simulink model "LQR_simulation"  (R2023a)
settings: Solver=FixedStepAuto  StartTime=0.0  StopTime=100  FixedStep=out_rate  RelTol=1e-3
InitFcn:
  | LQR_init
values from neighbouring files (symbols this model uses):
  C = [1 0 0 0;     0 1 0 0]    [LQR_init.m]
  dt = 0.001    [LQR_init.m]
  dtheta_0_real = dtheta_0+std_dev.dtheta_0*rand(1,1)    [LQR_init.m]
  dz_0_real = dz_0+std_dev.dz_0*randn(1,1)    [LQR_init.m]
  fa_w = 0    [LQR_init.m]
  fm_w = s_param.g*s_param.m    [LQR_init.m]
  K_a_lqr = - lqr(A_a,B_a,Q_a_lqr,R_a_lqr)    [LQR_init.m]
  K_lqr = - lqr(A,B,Q_lqr,R_lqr)    [LQR_init.m]
  Km1 = 1.1    [LQR_init.m]
  Km1_real = Km1 + std_dev_Km*randn(1,1)    [LQR_init.m]
  Km2 = 1.1    [LQR_init.m]
  Km2_real = Km2 + std_dev_Km*randn(1,1)    [LQR_init.m]
  m_treshold = 5    [LQR_init.m]
  out_rate = 0.001    [LQR_init.m]
  P_0 = blkdiag(std_dev.z_0^2, std_dev.theta_0^2, std_dev.dz_0^2, std_dev.dtheta_0^2)    [LQR_init.m]
  Q = blkdiag(std_dev.fm^2, std_dev.fa^2)    [LQR_init.m]
  R = blkdiag(std_dev.y1^2, std_dev.y2^2)    [LQR_init.m]
  T1 = 0.05    [LQR_init.m]
  T1_real = T1 + std_dev_T*randn(1,1)    [LQR_init.m]
  T2 = 0.15    [LQR_init.m]
  T2_real = T2 + std_dev_T*randn(1,1)    [LQR_init.m]
  theta_0_real = theta_0+std_dev.theta_0*randn(1,1)    [LQR_init.m]
  theta_w = 0    [LQR_init.m]
  Tm1 = 1    [LQR_init.m]
  Tm1_real = Tm1 + std_dev_Tm*randn(1,1)    [LQR_init.m]
  Tm2 = 1    [LQR_init.m]
  Tm2_real = Tm2 + std_dev_Tm*randn(1,1)    [LQR_init.m]
  U_mean = [0; 0]    [LQR_init.m]
  x_0 = [z_0; theta_0; dz_0; dtheta_0]    [LQR_init.m]
  x_a_w = [0;0;x_w]    [LQR_init.m]
  x_w = [z_w; theta_w; dz_w; dtheta_w]    [LQR_init.m]
  z_0_real = z_0+std_dev.z_0*randn(1,1)    [LQR_init.m]
  z_w = 400    [LQR_init.m]
undefined symbols (not defined in the file or in its folder): Kf, s_param, std_dev, Ts
libraries: simulink x4
settings Model: Creator=franc  LastModifiedBy=rvitt

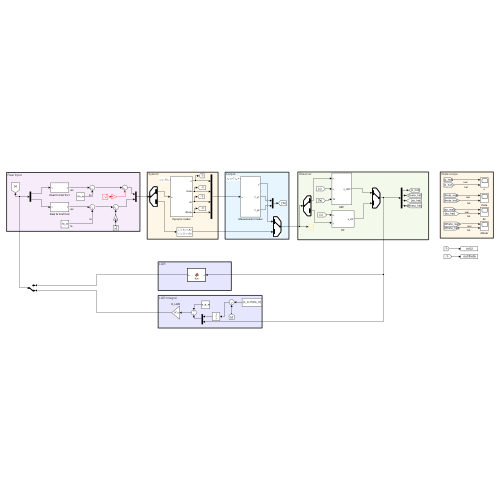
[thumbnail: Simulink's stored preview of the top-level diagram]
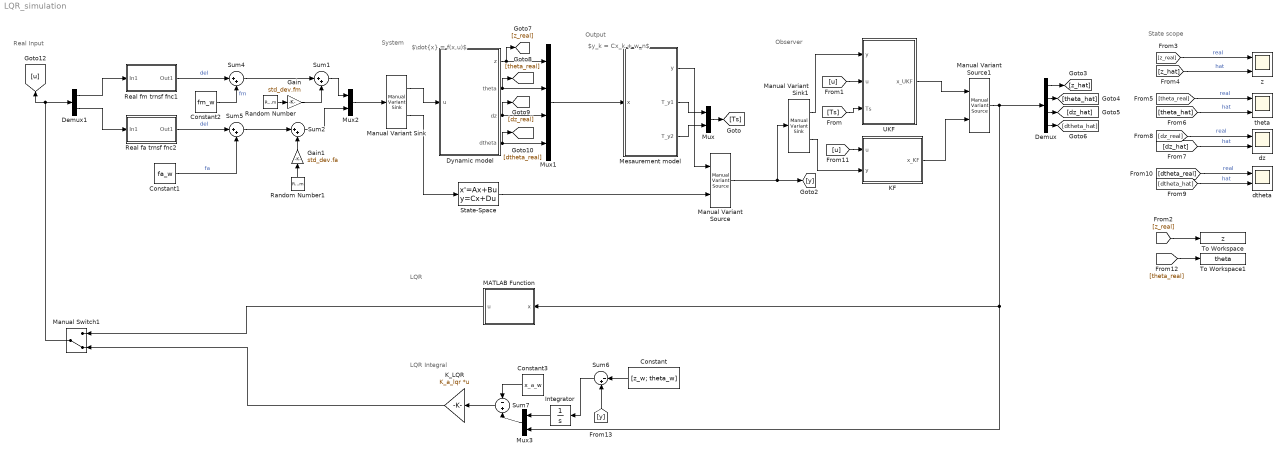
== system LQR_simulation ==
  note: State scope
  note: LQR Integral
  note: LQR
  note: Real Input
  note: Observer
  note: $y_k = Cx_k + w_n$
  note: Output
  note: $\dot{x} = f(x,u)$
  note: System
  Constant : Constant  Value=[z_w; theta_w]
  Constant1 : Constant  Value=fa_w
  Constant2 : Constant  Value=fm_w
  Constant3 : Constant  Value=x_a_w
  Demux : Demux
  Demux1 : Demux  Outputs=2
  Dynamic model : Subsystem
  Gain : Gain  Gain=std_dev.fm
  Gain1 : Gain  Gain=std_dev.fa
  Integrator : Integrator
  KF : Subsystem
  K_LQR : Gain  Gain=K_a_lqr  Multiplication=Matrix(K*u)
  MATLAB Function : MATLAB Function  TreatAsAtomicUnit=on
  Manual Variant Sink : simulink/Signal Routing/Manual Variant Sink  NumChoices=2  LabelModeActiveChoice=V_1
  Manual Variant Sink1 : simulink/Signal Routing/Manual Variant Sink  NumChoices=2  LabelModeActiveChoice=V_1
  Manual Variant Source : simulink/Signal Routing/Manual Variant Source  NumChoices=2  LabelModeActiveChoice=V_1
  Manual Variant Source1 : simulink/Signal Routing/Manual Variant Source  NumChoices=2  LabelModeActiveChoice=V_1
  Manual Switch1 : ManualSwitch  CurrentSetting=0
  Mesaurement model : Subsystem
  Mux : Mux  Inputs=2
  Mux1 : Mux
  Mux2 : Mux  Inputs=2
  Mux3 : Mux  Inputs=2
  Random Number : RandomNumber  SampleTime=out_rate
  Random Number1 : RandomNumber  SampleTime=out_rate
  Real fa trnsf fnc2 : Subsystem
  Real fm trnsf fnc1 : Subsystem
  State-Space : StateSpace  InitialCondition=0
  Sum{1..2,4..5} (4 alike) : Sum  Inputs=|++
  Sum6 : Sum  Inputs=|-+
  Sum7 : Sum  Inputs=-|+
  To Workspace : ToWorkspace  VariableName=z  SaveFormat=Timeseries  SampleTime=-1
  To Workspace1 : ToWorkspace  VariableName=theta  SaveFormat=Timeseries  SampleTime=-1
  UKF : Subsystem
  dtheta : Scope  NumInputPorts=2
  dz : Scope  NumInputPorts=2
  theta : Scope  NumInputPorts=2
  z : Scope  NumInputPorts=2
  wires:
  Mesaurement model/2(T_y1) -> Mux/1
  Mesaurement model/3(T_y2) -> Mux/2
  Mux/1 -> [Ts]
  [u] -> UKF/2(u)
  [Ts] -> UKF/3(Ts)
  UKF/1(x_UKF) -> Manual Variant Source1/1
  [z_real] -> z/1  "real"
  [z_hat] -> z/2  "hat"
  [theta_real] -> theta/1  "real"
  [theta_hat] -> theta/2  "hat"
  [dz_hat] -> dz/2  "hat"
  [dz_real] -> dz/1  "real"
  [dtheta_hat] -> dtheta/2  "hat"
  [dtheta_real] -> dtheta/1  "real"
  Mux1/1 -> Mesaurement model/1(x)
  Dynamic model/1(z) -> [z_real], Mux1/1
  Dynamic model/2(theta) -> Mux1/2, [theta_real]
  Dynamic model/3(dz) -> Mux1/3, [dz_real]
  Dynamic model/4(dtheta) -> Mux1/4, [dtheta_real]
  [u] -> KF/1(u)
  KF/1(x_KF) -> Manual Variant Source1/2
  Manual Variant Source1/1 -> MATLAB Function/1(x), Mux3/2, Demux/1
  Demux/1 -> [z_hat]
  Demux/2 -> [theta_hat]
  Demux/3 -> [dz_hat]
  Demux/4 -> [dtheta_hat]
  MATLAB Function/1(u) -> Manual Switch1/1
  Demux1/1 -> Real fm trnsf fnc1/1(In1)
  Sum1/1 -> Mux2/1
  Sum2/1 -> Mux2/2
  Gain/1 -> Sum1/2
  Gain1/1 -> Sum2/2
  Random Number/1 -> Gain/1
  Random Number1/1 -> Gain1/1
  Demux1/2 -> Real fa trnsf fnc2/1(In1)
  Real fm trnsf fnc1/1(Out1) -> Sum4/1  "del"
  Real fa trnsf fnc2/1(Out1) -> Sum5/1  "del"
  Sum4/1 -> Sum1/1
  Sum5/1 -> Sum2/1
  Constant2/1 -> Sum4/2  "fm"
  Constant1/1 -> Sum5/2  "fa"
  Manual Switch1/1 -> Demux1/1, [u]
  Constant/1 -> Sum6/1
  Mux3/1 -> Sum7/2
  Integrator/1 -> Mux3/1
  Sum6/1 -> Integrator/1
  [y] -> Sum6/2
  Mux2/1 -> Manual Variant Sink/1
  Manual Variant Sink/1 -> Dynamic model/1(u)
  Manual Variant Sink/2 -> State-Space/1
  Manual Variant Source/1 -> [y], Manual Variant Sink1/1
  Mesaurement model/1(y) -> Manual Variant Source/1
  State-Space/1 -> Manual Variant Source/2
  Manual Variant Sink1/1 -> UKF/1(y)
  Manual Variant Sink1/2 -> KF/2(y)
  Constant3/1 -> Sum7/1
  Sum7/1 -> K_LQR/1
  K_LQR/1 -> Manual Switch1/2
  [z_real] -> To Workspace/1
  [theta_real] -> To Workspace1/1

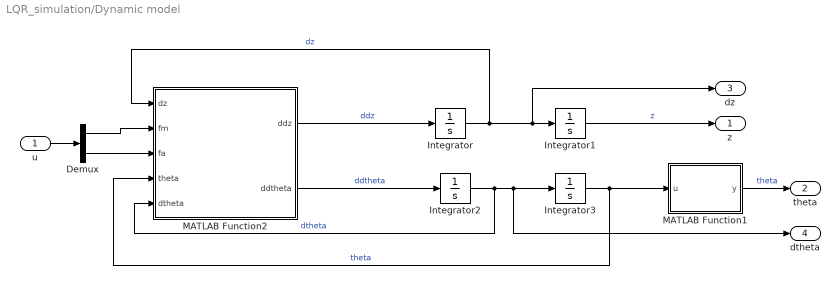
== system LQR_simulation/Dynamic model ==
  u : Inport
  Demux : Demux  Outputs=2
  Integrator : Integrator  InitialCondition=dz_0_real
  Integrator1 : Integrator  InitialCondition=z_0_real
  Integrator2 : Integrator  InitialCondition=dtheta_0_real
  Integrator3 : Integrator  InitialCondition=theta_0_real
  MATLAB Function1 : MATLAB Function  TreatAsAtomicUnit=on
  MATLAB Function2 : MATLAB Function  TreatAsAtomicUnit=on
  z : Outport
  theta : Outport  Port=2
  dz : Outport  Port=3
  dtheta : Outport  Port=4
  wires:
  Integrator3/1 -> MATLAB Function2/4(theta), MATLAB Function1/1(u)  "theta"
  Integrator2/1 -> dtheta/1, Integrator3/1, MATLAB Function2/5(dtheta)  "dtheta"
  MATLAB Function1/1(y) -> theta/1  "theta"
  Integrator1/1 -> z/1  "z"
  MATLAB Function2/2(ddtheta) -> Integrator2/1  "ddtheta"
  MATLAB Function2/1(ddz) -> Integrator/1  "ddz"
  Integrator/1 -> dz/1, Integrator1/1, MATLAB Function2/1(dz)  "dz"
  u/1 -> Demux/1
  Demux/2 -> MATLAB Function2/3(fa)
  Demux/1 -> MATLAB Function2/2(fm)

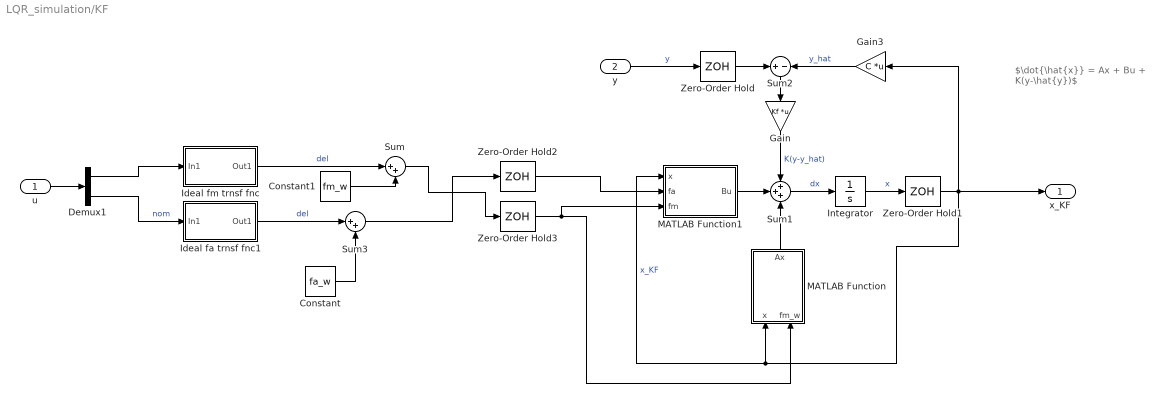
== system LQR_simulation/KF ==
  note: $\dot{\hat{x}} = Ax + Bu + K(y-\hat{y})$
  u : Inport
  y : Inport  Port=2
  Constant : Constant  Value=fa_w
  Constant1 : Constant  Value=fm_w
  Demux1 : Demux  Outputs=2
  Gain : Gain  Gain=Kf  Multiplication=Matrix(K*u)
  Gain3 : Gain  Gain=C  Multiplication=Matrix(K*u)
  Ideal fa trnsf fnc1 : Subsystem
  Ideal fm trnsf fnc : Subsystem
  Integrator : Integrator  InitialCondition=x_0
  MATLAB Function : MATLAB Function  TreatAsAtomicUnit=on
  MATLAB Function1 : MATLAB Function  TreatAsAtomicUnit=on
  Sum : Sum  Inputs=|++
  Sum1 : Sum  Inputs=+++
  Sum2 : Sum  Inputs=+|-
  Sum3 : Sum  Inputs=|++
  Zero-Order Hold{,1..3} (4 alike) : ZeroOrderHold  SampleTime=dt
  x_KF : Outport
  wires:
  y/1 -> Zero-Order Hold/1  "y"
  u/1 -> Demux1/1
  Gain3/1 -> Sum2/2  "y_hat"
  Sum1/1 -> Integrator/1  "dx"
  Sum2/1 -> Gain/1
  Gain/1 -> Sum1/1  "K(y-y_hat)"
  MATLAB Function1/1(Bu) -> Sum1/2
  Zero-Order Hold/1 -> Sum2/1
  Zero-Order Hold1/1 -> MATLAB Function1/1(x), MATLAB Function/1(x), Gain3/1, x_KF/1  "x_KF"
  Integrator/1 -> Zero-Order Hold1/1  "x"
  MATLAB Function/1(Ax) -> Sum1/3
  Zero-Order Hold2/1 -> MATLAB Function1/2(fa)
  Sum/1 -> Zero-Order Hold3/1
  Zero-Order Hold3/1 -> MATLAB Function1/3(fm), MATLAB Function/2(fm_w)
  Ideal fm trnsf fnc/1(Out1) -> Sum/1  "del"
  Constant1/1 -> Sum/2
  Demux1/1 -> Ideal fm trnsf fnc/1(In1)
  Ideal fa trnsf fnc1/1(Out1) -> Sum3/1  "del"
  Demux1/2 -> Ideal fa trnsf fnc1/1(In1)  "nom"
  Sum3/1 -> Zero-Order Hold2/1
  Constant/1 -> Sum3/2

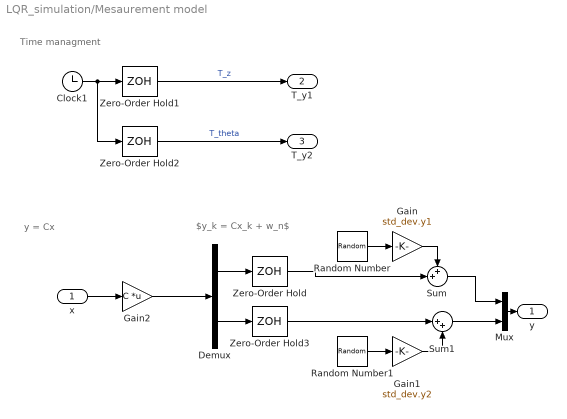
== system LQR_simulation/Mesaurement model ==
  note: $y_k = Cx_k + w_n$
  note: y = Cx
  note: Time managment
  x : Inport
  Clock1 : Clock
  Demux : Demux  Outputs=2
  Gain : Gain  Gain=std_dev.y1
  Gain1 : Gain  Gain=std_dev.y2
  Gain2 : Gain  Gain=C  Multiplication=Matrix(K*u)
  Mux : Mux  Inputs=2
  Random Number : RandomNumber  SampleTime=Ts.y1
  Random Number1 : RandomNumber  SampleTime=Ts.y2
  Sum : Sum  Inputs=++|
  Sum1 : Sum  Inputs=|++
  Zero-Order Hold : ZeroOrderHold  SampleTime=Ts.y1
  Zero-Order Hold1 : ZeroOrderHold  SampleTime=Ts.y1
  Zero-Order Hold2 : ZeroOrderHold  SampleTime=Ts.y2
  Zero-Order Hold3 : ZeroOrderHold  SampleTime=Ts.y2
  y : Outport
  T_y1 : Outport  Port=2
  T_y2 : Outport  Port=3
  wires:
  Demux/1 -> Zero-Order Hold/1
  Gain1/1 -> Sum1/2
  Random Number1/1 -> Gain1/1
  Demux/2 -> Zero-Order Hold3/1
  Gain/1 -> Sum/1
  Clock1/1 -> Zero-Order Hold2/1, Zero-Order Hold1/1
  Zero-Order Hold2/1 -> T_y2/1  "T_theta"
  Sum1/1 -> Mux/2
  Zero-Order Hold1/1 -> T_y1/1  "T_z"
  Sum/1 -> Mux/1
  x/1 -> Gain2/1
  Gain2/1 -> Demux/1
  Random Number/1 -> Gain/1
  Zero-Order Hold/1 -> Sum/2
  Zero-Order Hold3/1 -> Sum1/1
  Mux/1 -> y/1

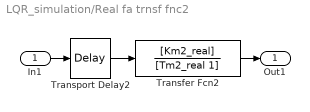
== system LQR_simulation/Real fa trnsf fnc2 ==
  In1 : Inport
  Transfer Fcn2 : TransferFcn  Numerator=[Km2_real]  Denominator=[Tm2_real 1]
  Transport Delay2 : TransportDelay  DelayTime=T2_real
  Out1 : Outport
  wires:
  Transport Delay2/1 -> Transfer Fcn2/1
  Transfer Fcn2/1 -> Out1/1
  In1/1 -> Transport Delay2/1

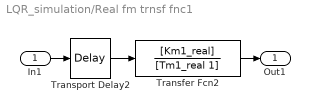
== system LQR_simulation/Real fm trnsf fnc1 ==
  In1 : Inport
  Transfer Fcn2 : TransferFcn  Numerator=[Km1_real]  Denominator=[Tm1_real 1]
  Transport Delay2 : TransportDelay  DelayTime=T1_real
  Out1 : Outport
  wires:
  In1/1 -> Transport Delay2/1
  Transfer Fcn2/1 -> Out1/1
  Transport Delay2/1 -> Transfer Fcn2/1

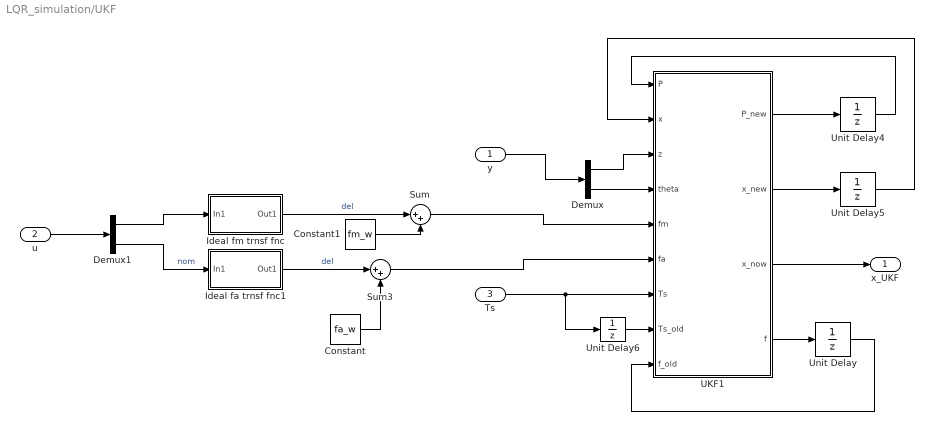
== system LQR_simulation/UKF ==
  y : Inport
  u : Inport  Port=2
  Ts : Inport  Port=3
  Constant : Constant  Value=fa_w
  Constant1 : Constant  Value=fm_w
  Demux : Demux  Outputs=2
  Demux1 : Demux  Outputs=2
  Ideal fa trnsf fnc1 : Subsystem
  Ideal fm trnsf fnc : Subsystem
  Sum : Sum  Inputs=|++
  Sum3 : Sum  Inputs=|++
  UKF1 : MATLAB Function  TreatAsAtomicUnit=on  SystemSampleTime=dt
  Unit Delay : UnitDelay  InitialCondition=[1; 1]  SampleTime=-1  HasFrameUpgradeWarning=on
  Unit Delay4 : UnitDelay  InitialCondition=P_0  SampleTime=-1  HasFrameUpgradeWarning=on
  Unit Delay5 : UnitDelay  InitialCondition=x_0  SampleTime=-1  HasFrameUpgradeWarning=on
  Unit Delay6 : UnitDelay  SampleTime=dt  HasFrameUpgradeWarning=on
  x_UKF : Outport
  wires:
  Unit Delay4/1 -> UKF1/1(P)
  UKF1/4(f) -> Unit Delay/1
  Unit Delay5/1 -> UKF1/2(x)
  Unit Delay/1 -> UKF1/9(f_old)
  Unit Delay6/1 -> UKF1/8(Ts_old)
  UKF1/1(P_new) -> Unit Delay4/1
  UKF1/2(x_new) -> Unit Delay5/1
  u/1 -> Demux1/1
  Ts/1 -> Unit Delay6/1, UKF1/7(Ts)
  UKF1/3(x_now) -> x_UKF/1
  Demux/1 -> UKF1/3(z)
  Demux/2 -> UKF1/4(theta)
  Demux1/1 -> Ideal fm trnsf fnc/1(In1)
  Ideal fa trnsf fnc1/1(Out1) -> Sum3/1  "del"
  Demux1/2 -> Ideal fa trnsf fnc1/1(In1)  "nom"
  Sum3/1 -> UKF1/6(fa)
  Constant/1 -> Sum3/2
  Ideal fm trnsf fnc/1(Out1) -> Sum/1  "del"
  Sum/1 -> UKF1/5(fm)
  y/1 -> Demux/1
  Constant1/1 -> Sum/2

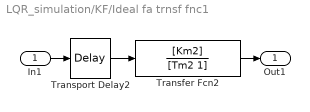
== system LQR_simulation/KF/Ideal fa trnsf fnc1 ==
  In1 : Inport
  Transfer Fcn2 : TransferFcn  Numerator=[Km2]  Denominator=[Tm2 1]
  Transport Delay2 : TransportDelay  DelayTime=T2
  Out1 : Outport
  wires:
  In1/1 -> Transport Delay2/1
  Transfer Fcn2/1 -> Out1/1
  Transport Delay2/1 -> Transfer Fcn2/1

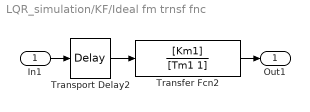
== system LQR_simulation/KF/Ideal fm trnsf fnc ==
  In1 : Inport
  Transfer Fcn2 : TransferFcn  Numerator=[Km1]  Denominator=[Tm1 1]
  Transport Delay2 : TransportDelay  DelayTime=T1
  Out1 : Outport
  wires:
  Transport Delay2/1 -> Transfer Fcn2/1
  Transfer Fcn2/1 -> Out1/1
  In1/1 -> Transport Delay2/1

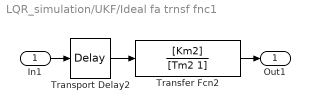
== system LQR_simulation/UKF/Ideal fa trnsf fnc1 ==
  In1 : Inport
  Transfer Fcn2 : TransferFcn  Numerator=[Km2]  Denominator=[Tm2 1]
  Transport Delay2 : TransportDelay  DelayTime=T2
  Out1 : Outport
  wires:
  In1/1 -> Transport Delay2/1
  Transfer Fcn2/1 -> Out1/1
  Transport Delay2/1 -> Transfer Fcn2/1

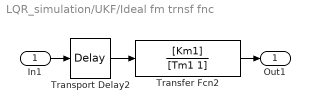
== system LQR_simulation/UKF/Ideal fm trnsf fnc ==
  In1 : Inport
  Transfer Fcn2 : TransferFcn  Numerator=[Km1]  Denominator=[Tm1 1]
  Transport Delay2 : TransportDelay  DelayTime=T1
  Out1 : Outport
  wires:
  Transport Delay2/1 -> Transfer Fcn2/1
  Transfer Fcn2/1 -> Out1/1
  In1/1 -> Transport Delay2/1

== matlab function LQR_simulation/Dynamic model/MATLAB Function1 ==
  data: u input; y output
function y = fcn(u)

y = atan2(sin(u), cos(u));
end

== matlab function LQR_simulation/KF/MATLAB Function ==
  data: x input; Ax output; fm_w input; s_param parameter
function Ax = fcn(x, fm_w, s_param)

theta_w = x(2);

A = [0 0 1 0;...
    0 0 0 1;...
    0 -fm_w*sin(theta_w)/s_param.m -s_param.b/s_param.m 0;...
    0 0 0 -s_param.b/s_param.J];


Ax = A*x;

== matlab function LQR_simulation/Dynamic model/MATLAB Function2 ==
  data: dz input; fm input; fa input; ddz output; ddtheta output; theta input; dtheta input; s_param parameter
function [ddz, ddtheta] = fcn(dz, fm, fa, theta, dtheta, s_param)

% Rename params
J = s_param.J;     
m = s_param.m;     
b = s_param.b;      
beta = s_param.beta;    
g = s_param.g;     
l = s_param.l;   

%% Dynamic equations

ddz = -b/m * dz + fm/m * cos(theta) -g;
ddtheta = -beta/J * dtheta + 2 * l/J * fa;

end

== matlab function LQR_simulation/MATLAB Function ==
  data: x input; u output; K_lqr parameter; x_w parameter
function u = fcn(x, K_lqr, x_w)

u = K_lqr*(x - x_w);
end

== matlab function LQR_simulation/KF/MATLAB Function1 ==
  data: x input; Bu output; fa input; fm input; s_param parameter
function Bu = fcn(x, fa, fm, s_param)

theta_w = x(2);

u = [fm;fa];

B = [0 0;...
    0 0;...
    cos(theta_w)/s_param.m 0;
    0 2*s_param.l/s_param.J]; 

Bu = B*u;

== matlab function LQR_simulation/UKF/UKF1 ==
  data: P_new output; x_new output; x_now output; P input; x input; z input; theta input; fm input; fa input; s_param parameter; R parameter; dt parameter; Q parameter; U_mean parameter; Ts input; Ts_old input; f_old input; f output; m_treshold parameter; C parameter
function [P_new, x_new, x_now, f] = UKF(P, x, z, theta, fm, fa, s_param, R, dt, Q, U_mean,Ts, Ts_old, f_old, m_treshold, C)
%% UKF algorithm

%% Correction

f = f_old;

% Flag refreshing
for i = 1:2
    if Ts(i) > Ts_old(i)
        f(i) = 1;
    end
end

y = [z; theta];

% Compute innovation
e = y - C*x;
e(2) = atan2( sin( e(2) ), cos( e(2) ) );

% Compute covariance innovation
S = C*P*transpose(C) + R;
inv_S = pinv(S);

% Compute Cross Covariance
cross_cov = P*transpose(C);

% Compute Mahalanobis distance
mahalanobis_distance = sqrt(e'*inv_S*e);

% Gain matrix init
L = zeros(size(x,1),size(y,1));

% Management of conditions for correction
for i = 1:2
    if ( f(i) ) && ( mahalanobis_distance < m_treshold )
        L(:,i) = cross_cov*inv_S(:,i);
        f(i) = 0;
    else
        L(:,i) = zeros(size(x,1),1);
        f(i) = f_old(i);
    end
end

x_now = x + L*e;                  
P_now = P - L*S*transpose(L);

%% Prediction
[x_new, P_new] = UT_F(x_now, P_now, dt, fm, fa, s_param, Q, U_mean);
end
